simulink model "gm_DUC"  (R2024b)
settings: Solver=FixedStepDiscrete  StartTime=0.0  StopTime=0.008  FixedStep=8.33333333333333e-09  RelTol=1e-3
undefined symbols (not defined in the file or in its folder): cicComp_1, cicComp_2, fs, hb1, hb2, N1_cycle, N2_cycle, N_cic1_itp, N_cic2_itp, phInc_base_1, phInc_base_2, up_L
libraries: dsphdlfiltering2 x4, dsphdlsigops2 x3, dspmlti4 x2, hdlsllib x2, simulink x1
settings Model: Creator=31651  LastModifiedBy=31651
settings OptimizationCC: BlockReduction=off  ConditionallyExecuteInputs=off
settings DebuggingCC: InheritedTsInSrcMsg=none  SingleTaskRateTransMsg=error
settings RTWCC: GPUComputeCapability=3.5

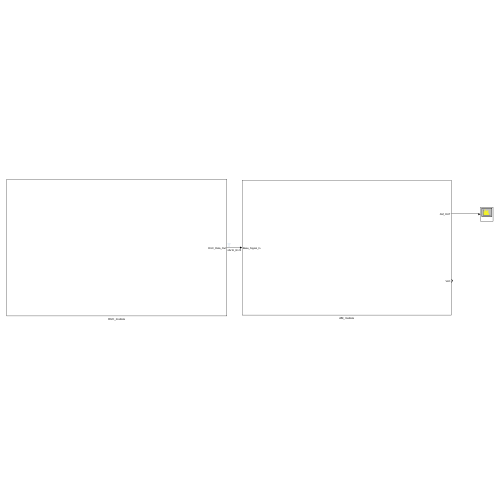
[thumbnail: Simulink's stored preview of the top-level diagram]
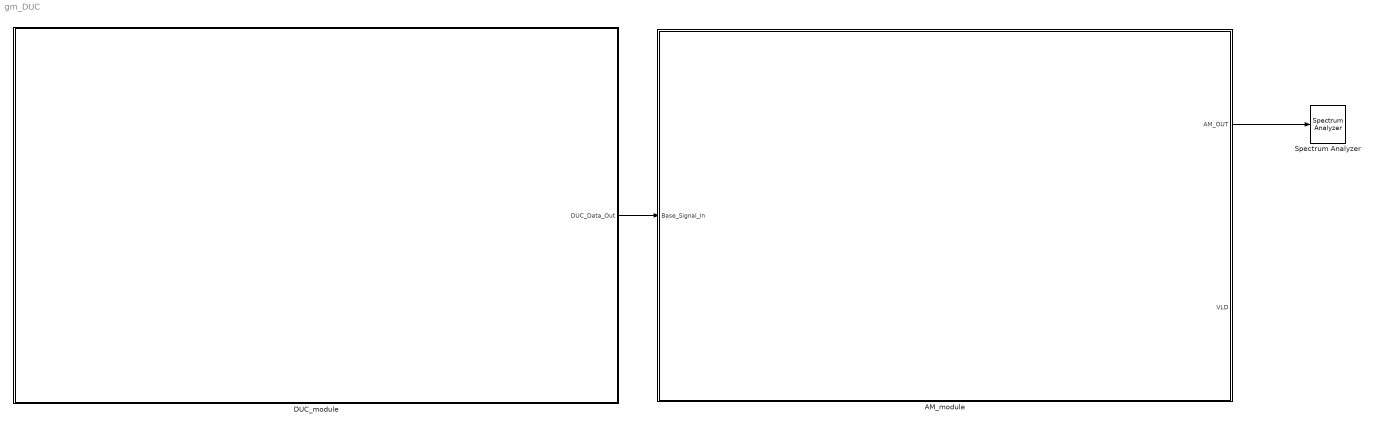
== system gm_DUC ==
  AM_module : Subsystem
  DUC_module : Subsystem
  Spectrum Analyzer : SpectrumAnalyzer  WindowPosition=[811.000000,458.000000,800.000000,500.000000,]  Visible=on  ScopeFrameLocation=window  WindowInvariantSamplesPerUpdate=on  YLimits=[-87.50865668,31.61502968]
  wires:
  AM_module/1(AM_OUT) -> Spectrum Analyzer/1
  DUC_module/1(DUC_Data_Out) -> AM_module/1(Base_Signal_In)

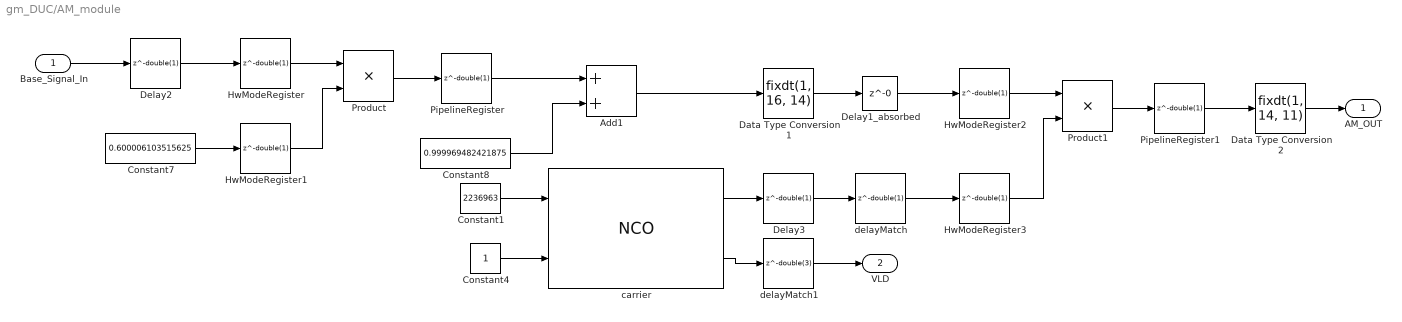
== system gm_DUC/AM_module ==
  Base_Signal_In : Inport  OutDataTypeStr=fixdt(1, 16, 15)  PortDimensions=1  SampleTime=8.33333333333333e-09
  Add1 : Sum  OutDataTypeStr=fixdt(1, 32, 30)  AccumDataTypeStr=fixdt(1, 32, 30)  SampleTime=8.33333333333333e-09
  Constant1 : Constant  Value=2236963  OutDataTypeStr=uint32  SampleTime=8.33333333333333e-09
  Constant4 : Constant  OutDataTypeStr=boolean  SampleTime=8.33333333333333e-09
  Constant7 : Constant  Value=0.600006103515625  OutDataTypeStr=fixdt(1, 16, 15)  SampleTime=8.33333333333333e-09
  Constant8 : Constant  Value=0.999969482421875  OutDataTypeStr=fixdt(1, 16, 15)  SampleTime=8.33333333333333e-09
  Data Type Conversion1 : DataTypeConversion  OutDataTypeStr=fixdt(1, 16, 14)  SampleTime=8.33333333333333e-09  RndMeth=Floor
  Data Type Conversion2 : DataTypeConversion  OutDataTypeStr=fixdt(1, 14, 11)  SampleTime=8.33333333333333e-09  RndMeth=Floor
  Delay1_absorbed : Delay  DelayLength=0
  Delay2 : Delay  DelayLength=double(1)  InitialCondition=0  SampleTime=8.33333333333333e-09
  Delay3 : Delay  DelayLength=double(1)  InitialCondition=0  SampleTime=8.33333333333333e-09
  HwModeRegister{,1..3} (4 alike) : Delay  DelayLength=double(1)  InitialCondition=0  SampleTime=8.33333333333333e-09
  PipelineRegister : Delay  DelayLength=double(1)  InitialCondition=0  SampleTime=8.33333333333333e-09
  PipelineRegister1 : Delay  DelayLength=double(1)  InitialCondition=0  SampleTime=8.33333333333333e-09
  Product : Product  Inputs=**  OutDataTypeStr=fixdt(1, 32, 30)  SampleTime=8.33333333333333e-09
  Product1 : Product  Inputs=**  OutDataTypeStr=fixdt(1, 32, 29)  SampleTime=8.33333333333333e-09
  carrier : dsphdlsigops2/NCO  PhaseIncrementSource=Input port  PhaseIncrement=100  PhaseOffsetSource=Property  PhaseOffset=0  DitherSource=Property  NumDitherBits=ditherBits  SamplesPerFrame=1  LUTCompress=off  ResetAction=off  Waveform=Sine  PhasePort=off  SimulateUsing=Code generation  AccumulatorWL=Nnco  PhaseQuantization=on  NumQuantizerAccumulatorBits=Q  OutputDataType=Binary point scaling  OutputWL=16  OutputFL=15
      settings: LibrarySourceBlock=dsphdlsrcs2/NCO
  delayMatch : Delay  DelayLength=double(1)  InitialCondition=0  SampleTime=8.33333333333333e-09
  delayMatch1 : Delay  DelayLength=double(3)  InitialCondition=0  SampleTime=8.33333333333333e-09
  AM_OUT : Outport  SampleTime=8.33333333333333e-09
  VLD : Outport  Port=2  SampleTime=8.33333333333333e-09
  wires:
  Base_Signal_In/1 -> Delay2/1
  HwModeRegister1/1 -> Product/2
  Delay2/1 -> HwModeRegister/1
  HwModeRegister/1 -> Product/1
  Product/1 -> PipelineRegister/1
  Data Type Conversion1/1 -> Delay1_absorbed/1
  Constant7/1 -> HwModeRegister1/1
  PipelineRegister/1 -> Add1/1
  Constant8/1 -> Add1/2
  Constant1/1 -> carrier/1
  Constant4/1 -> carrier/2
  Add1/1 -> Data Type Conversion1/1
  carrier/1 -> Delay3/1
  carrier/2 -> delayMatch1/1
  Delay3/1 -> delayMatch/1
  delayMatch1/1 -> VLD/1
  Delay1_absorbed/1 -> HwModeRegister2/1
  delayMatch/1 -> HwModeRegister3/1
  HwModeRegister2/1 -> Product1/1
  HwModeRegister3/1 -> Product1/2
  Product1/1 -> PipelineRegister1/1
  PipelineRegister1/1 -> Data Type Conversion2/1
  Data Type Conversion2/1 -> AM_OUT/1

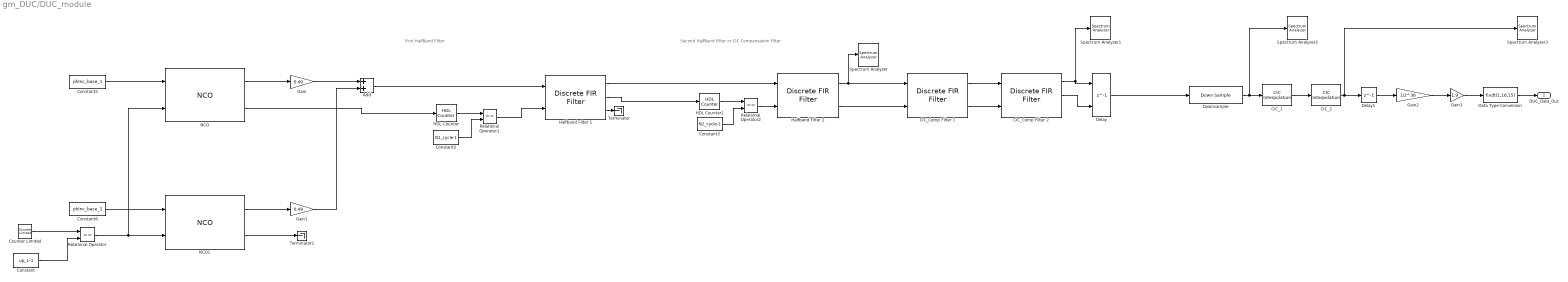
== system gm_DUC/DUC_module ==
  note: First HalfBand Filter
  note: Second HalfBand Filter or CIC Compensation Filter
  Add : Sum
  CIC_1 : dspmlti4/CIC Interpolation  filtFrom=Dialog parameters  filtobj=Hm_interp  ftype=Interpolator  R=N_cic1_itp  M=1  N=5  filterInternals=Minimum section word lengths  BPS=[16 16 16 16]  FLPS=0  outputWordLength=16  outputFracLength=0  launchFVT=off  framing=Allow multirate processing  OutputFrames=off
  CIC_2 : dspmlti4/CIC Interpolation  filtFrom=Dialog parameters  filtobj=Hm_interp  ftype=Interpolator  R=N_cic2_itp  M=1  N=5  filterInternals=Minimum section word lengths  BPS=[16 16 16 16]  FLPS=0  outputWordLength=16  outputFracLength=0  launchFVT=off  framing=Allow multirate processing  OutputFrames=off
  CIC_Comp Filter 1 : dsphdlfiltering2/Discrete FIR Filter  NumeratorSource=Property  Numerator=cicComp_1.Numerator  NumeratorPrototype=[]  FilterStructure=Direct form systolic  SerializationOption=Minimum number of cycles between valid input samples  NumCycles=2  NumberOfMultipliers=2  SimulateUsing=Code generation  roundingMode=Floor  overflowMode=off  CoefficientsDataTypeStr=Inherit: Same word length as input  OutputDataTypeStr=fixdt(1,16,15)  ResetInputPort=off  HDLGlobalReset=off  CoeffMultiplier=Multiplier  UseMultForPow2Coeff=on
  CIC_Comp Filter 2 : dsphdlfiltering2/Discrete FIR Filter  NumeratorSource=Property  Numerator=cicComp_2.Numerator  NumeratorPrototype=[]  FilterStructure=Partly serial systolic  SerializationOption=Minimum number of cycles between valid input samples  NumCycles=2  NumberOfMultipliers=2  SimulateUsing=Code generation  roundingMode=Floor  overflowMode=off  CoefficientsDataTypeStr=Inherit: Same word length as input  OutputDataTypeStr=fixdt(1,16,15)  ResetInputPort=off  HDLGlobalReset=off  CoeffMultiplier=Multiplier  UseMultForPow2Coeff=on
  Constant : Constant  Value=up_L-1  OutDataTypeStr=uint16  SampleTime=1/fs
  Constant2 : Constant  Value=N1_cycle-1  OutDataTypeStr=uint16  SampleTime=1/fs
  Constant3 : Constant  Value=N2_cycle-1  OutDataTypeStr=uint16  SampleTime=1/fs
  Constant5 : Constant  Value=phInc_base_1  OutDataTypeStr=uint32  SampleTime=1/fs
  Constant6 : Constant  Value=phInc_base_2  OutDataTypeStr=uint32  SampleTime=1/fs
  Counter Limited : simulink/Sources/Counter Limited  uplimit=up_L-1  tsamp=1/fs
  Data Type Conversion : DataTypeConversion  OutDataTypeStr=fixdt(1,16,15)  ConvertRealWorld=Stored Integer (SI)  SaturateOnIntegerOverflow=off  RndMeth=Floor
  Delay : Delay  DelayLength=1  ShowEnablePort=on
      settings: InputPortMap=u0,e6
  Delay1 : Delay  DelayLength=1
  Downsample : DownSample  N=N2_cycle  RateOptions=Allow multirate processing
  Gain : Gain  Gain=0.49
  Gain1 : Gain  Gain=0.49
  Gain2 : Gain  Gain=1/2^36  OutDataTypeStr=fixdt(1,16,14)
  Gain3 : Gain  Gain=1.9  OutDataTypeStr=fixdt(1,16,15)
  HDL Counter : hdlsllib/Sources/HDL Counter  CountType=Count limited  CountInit=0  CountStep=1  CountMax=N1_cycle-1  CountFromType=Initial value  CountFrom=0  CountResetPort=on  CountLoadPort=off  CountEnbPort=off  CountDirPort=off  CountHitOutputPort=off  CountDataType=Unsigned  CountWordLen=16  CountFracLen=0  CountSampTime=1
  HDL Counter1 : hdlsllib/Sources/HDL Counter  CountType=Count limited  CountInit=0  CountStep=1  CountMax=N2_cycle-1  CountFromType=Initial value  CountFrom=0  CountResetPort=on  CountLoadPort=off  CountEnbPort=off  CountDirPort=off  CountHitOutputPort=off  CountDataType=Unsigned  CountWordLen=16  CountFracLen=0  CountSampTime=1
  Halfband Filter 1 : dsphdlfiltering2/Discrete FIR Filter  NumeratorSource=Property  Numerator=hb1.Numerator  NumeratorPrototype=[]  FilterStructure=Partly serial systolic  SerializationOption=Minimum number of cycles between valid input samples  NumCycles=4  NumberOfMultipliers=2  SimulateUsing=Code generation  roundingMode=Floor  overflowMode=off  CoefficientsDataTypeStr=Inherit: Same word length as input  OutputDataTypeStr=fixdt(1,16,15)  ResetInputPort=off  HDLGlobalReset=off  CoeffMultiplier=Multiplier  UseMultForPow2Coeff=on
  Halfband Filter 2 : dsphdlfiltering2/Discrete FIR Filter  NumeratorSource=Property  Numerator=hb2.Numerator  NumeratorPrototype=[]  FilterStructure=Direct form systolic  SerializationOption=Minimum number of cycles between valid input samples  NumCycles=4  NumberOfMultipliers=2  SimulateUsing=Code generation  roundingMode=Floor  overflowMode=off  CoefficientsDataTypeStr=Inherit: Same word length as input  OutputDataTypeStr=fixdt(1,16,15)  ResetInputPort=off  HDLGlobalReset=off  CoeffMultiplier=Multiplier  UseMultForPow2Coeff=on
  NCO : dsphdlsigops2/NCO  PhaseIncrementSource=Input port  PhaseIncrement=100  PhaseOffsetSource=Property  PhaseOffset=0  DitherSource=Property  NumDitherBits=ditherBits  SamplesPerFrame=1  LUTCompress=off  ResetAction=off  Waveform=Sine  PhasePort=off  SimulateUsing=Code generation  AccumulatorWL=Nnco  PhaseQuantization=on  NumQuantizerAccumulatorBits=Q  OutputDataType=Binary point scaling  OutputWL=16  OutputFL=14
  NCO1 : dsphdlsigops2/NCO  PhaseIncrementSource=Input port  PhaseIncrement=100  PhaseOffsetSource=Property  PhaseOffset=0  DitherSource=Property  NumDitherBits=ditherBits  SamplesPerFrame=1  LUTCompress=off  ResetAction=off  Waveform=Sine  PhasePort=off  SimulateUsing=Code generation  AccumulatorWL=Nnco  PhaseQuantization=on  NumQuantizerAccumulatorBits=Q  OutputDataType=Binary point scaling  OutputWL=16  OutputFL=14
  Relational Operator : RelationalOperator  Operator===  OutDataTypeStr=boolean  RndMeth=Simplest  InputSameDT=off
  Relational Operator1 : RelationalOperator  Operator===  OutDataTypeStr=boolean  RndMeth=Simplest  InputSameDT=off
  Relational Operator2 : RelationalOperator  Operator===  OutDataTypeStr=boolean  RndMeth=Simplest  InputSameDT=off
  Spectrum Analyzer : SpectrumAnalyzer  WindowPosition=[1674.000000,795.000000,800.000000,500.000000,]  Visible=on  ScopeFrameLocation=window  WindowInvariantSamplesPerUpdate=on  Span=120000000  StartFrequency=-60000000  StopFrequency=60000000  YLimits=[-118.75683094,-31.36588238]
  Spectrum Analyzer1 : SpectrumAnalyzer  WindowPosition=[1571.000000,748.000000,800.000000,602.000000,]  Visible=on  ScopeFrameLocation=window  WindowInvariantSamplesPerUpdate=on  Span=120000000  StartFrequency=-60000000  StopFrequency=60000000  YLimits=[-126.82761037,-44.27246761]
  Spectrum Analyzer2 : SpectrumAnalyzer  WindowPosition=[1633.000000,187.000000,800.000000,500.000000,]  Visible=on  ScopeFrameLocation=window  WindowInvariantSamplesPerUpdate=on  Span=120000000  StartFrequency=-60000000  StopFrequency=60000000  YLimits=[-54.63000723,6.73072266]
  Spectrum Analyzer3 : SpectrumAnalyzer  WindowPosition=[1833.000000,-38.000000,800.000000,500.000000,]  Visible=on  ScopeFrameLocation=window  WindowInvariantSamplesPerUpdate=on  Span=120000000  StartFrequency=-60000000  StopFrequency=60000000  YLimits=[100.5157,238.3287]
  Terminator : Terminator
  Terminator1 : Terminator
  DUC_Data_Out : Outport
  wires:
  Delay1/1 -> Gain2/1
  CIC_2/1 -> Spectrum Analyzer3/1, Delay1/1
  Data Type Conversion/1 -> DUC_Data_Out/1
  Gain3/1 -> Data Type Conversion/1
  Gain2/1 -> Gain3/1
  CIC_1/1 -> CIC_2/1
  NCO1/2 -> Terminator1/1
  Halfband Filter 1/3 -> Terminator/1
  Constant3/1 -> Relational Operator2/2
  HDL Counter1/1 -> Relational Operator2/1
  Delay/1 -> Downsample/1
  Constant/1 -> Relational Operator/2
  Downsample/1 -> CIC_1/1, Spectrum Analyzer2/1
  CIC_Comp Filter 1/2 -> CIC_Comp Filter 2/2
  Halfband Filter 2/2 -> CIC_Comp Filter 1/2
  NCO/2 -> HDL Counter/1
  NCO1/1 -> Gain1/1
  Gain/1 -> Add/1
  Halfband Filter 1/2 -> HDL Counter1/1
  Add/1 -> Halfband Filter 1/1
  Constant6/1 -> NCO1/1
  Constant5/1 -> NCO/1
  HDL Counter/1 -> Relational Operator1/1
  Relational Operator1/1 -> Halfband Filter 1/2
  Counter Limited/1 -> Relational Operator/1
  Halfband Filter 2/1 -> Spectrum Analyzer/1, CIC_Comp Filter 1/1
  CIC_Comp Filter 1/1 -> CIC_Comp Filter 2/1
  CIC_Comp Filter 2/2 -> Delay/2
  Relational Operator/1 -> NCO1/2, NCO/2
  Gain1/1 -> Add/2
  NCO/1 -> Gain/1
  Relational Operator2/1 -> Halfband Filter 2/2
  CIC_Comp Filter 2/1 -> Spectrum Analyzer1/1, Delay/1
  Halfband Filter 1/1 -> Halfband Filter 2/1
  Constant2/1 -> Relational Operator1/2
